simulink library "LibraryFM"  (R2016b)
settings: Solver=VariableStepAuto  StartTime=0.0  StopTime=10.0  RelTol=1e-3
undefined symbols (not defined in the file or in its folder): ActuatorStruct, drivePeakCurrent, FM1, Lb, Lf, Lu, motorTorqueConstant, RobotStruct, sampleTime, transmissionRatio
undefined symbols (not defined in the file): JointAbsoluteEncoderCounts_rev
libraries: simulink x34, LibraryFM x13, VariousBlocksLibrary x4, dspstat3 x1, simulink_extras x1, FM_Library x1
(part 3 of 3)

== matlab function LibraryFM/ToActuator1/DriveEnableLogic/8_JointVelocityGuard/LPF Diff/MATLAB Function ==
  data: u input; freq input; y output; y_prev input; sampleTime parameter
function y = fcn(u,freq,y_prev,sampleTime)
tau = 1/(freq*2*pi);
a = sampleTime/(sampleTime + tau);
y = y_prev*(1-a) + a*u;

== matlab function LibraryFM/Subsystem3/visuomotor rotation1 ==
  data: xBound input; pos_ref output; yBound input; vel input; pos_ref_prev input; sampleTime parameter; vel_ref output
function [pos_ref, vel_ref] = rotation(xBound, yBound, vel, pos_ref_prev,sampleTime)

persistent velDir;

if isempty(velDir)
    velDir = [1;0]; % initial velocity
end

pos_ref_tmp = pos_ref_prev + velDir*vel*sampleTime;

% check for x boundary
if (pos_ref_tmp(1) > xBound)
    velDir = [0;1];
elseif (pos_ref_tmp(1) < -xBound)
    velDir = [0;-1];
elseif (pos_ref_tmp(2) > yBound)
    velDir = [-1;0];
elseif (pos_ref_tmp(2) < -yBound)
    velDir = [1;0];
end

% forward Euler integration
pos_ref = pos_ref_prev + velDir*vel*sampleTime;
vel_ref = velDir*vel;

end

== matlab function LibraryFM/visuomotor rotation ==
  data: x_home input; x input; y output; theta input; doRotation input
function y = fcn(x_home,x,theta,doRotation)

x = x - x_home;

if (doRotation)
    R = [cos(theta) -sin(theta); 
         sin(theta) cos(theta)];
    y = R*x;
else
    y = x;
end

y = y + x_home;

== matlab function LibraryFM/DriveEnableLogic1/8_JointVelocityGuard/LPF Diff/MATLAB Function ==
  data: u input; freq input; y output; y_prev input; sampleTime parameter
function y = fcn(u,freq,y_prev,sampleTime)
tau = 1/(freq*2*pi);
a = sampleTime/(sampleTime + tau);
y = y_prev*(1-a) + a*u;

== stateflow chart LibraryFM/DriveEnableLogic1/DriveEnableStateMachine ==
  state Off
    state Par1 [parallel]
      settings: executionOrder=1
      state KeepLatchValue
      state ResetLatchValue
        en:
        LatchDriveError_Rising = 0;
      (default) -> KeepLatchValue
      KeepLatchValue -> ResetLatchValue : [after(10,msec)]
    state Par2 [parallel]
      settings: executionOrder=2
      state Off_NoErrorReset
        en:
        ControlWord = uint16(6);
      state Off_ErrorReset
        en:
        ControlWord = uint16(128+6);
      (default) -> Off_NoErrorReset
      Off_NoErrorReset -> Off_ErrorReset : [UseActuator && ...
          | AutoResetErrorInterval_Off_ms~=0 && ...
          |  after(AutoResetErrorInterval_Off_ms, msec)]
      Off_ErrorReset -> Off_NoErrorReset : [after(10,msec)]
  note: This can be either of states:
      | NotReadyToSwitchOn
      | SwitchOnDisabled
      | Fault
      | ReadyToSwitchOn
  note: This chart here  resembles the relevant parts of the DS402 specification on state transitions. Note however that I do NOT check which state the system is in by investigating the value of the StatusWord. Instead, I just assume that everything works as it should.
      |
      | (This chart evolved from a programmatic state machine which also did not do this)
  state ReadyToSwitchOn
  note: During this transition: Reset any error
  state SwitchedOn
    en: LatchDriveError_Rising=1;
    ex: LatchDriveError_Rising=0;
  note: We use this state also to reset the DriveError display.
  state OperationEnabled
    en:DriveShouldBeEnabled=1;
    ex:DriveShouldBeEnabled=0;
    state OE_NoErrorReset
      en:
      ControlWord = uint16(15);
    state OE_ErrorReset
      en:
      ControlWord = uint16(128+15);
    OE_ErrorReset -> OE_NoErrorReset : [after(10,msec)]
    (default) -> OE_NoErrorReset
    OE_NoErrorReset -> OE_ErrorReset : [AutoResetErrorInterval_On_ms~=0 && ...
        |  after(AutoResetErrorInterval_On_ms, msec)]
  (default) -> Off : {ControlWord=uint16(6)}
  (junction 41) -> Off : {ControlWord=uint16(6); ...
      | LatchDriveError_Rising=1}
  (junction 40) -> (junction 41)
  Off -> ReadyToSwitchOn : [UseActuator && EnableRequest]{ControlWord = uint16(128+6)}
  OperationEnabled -> ReadyToSwitchOn [order 2] : [EnableRequest]{ControlWord=uint16(128+6)}
  ReadyToSwitchOn -> (junction 22) : [after(20,msec)]
  (junction 22) -> (junction 40) [order 2] : [DriveErrorIn]
  (junction 44) -> (junction 40)
  (junction 22) -> SwitchedOn [order 1] : [~DriveErrorIn]{ControlWord=uint16(7)}
  SwitchedOn -> (junction 44) [order 2] : [~UseActuator || ...
      | DriveErrorIn || ...
      | DisableRequest]
  (junction 45) -> (junction 44)
  SwitchedOn -> OperationEnabled [order 1] : [after(150,msec)]{ControlWord=uint16(15)}
  OperationEnabled -> (junction 45) [order 1] : [~UseActuator || ...
      | DriveErrorIn || ...
      | DisableRequest]
  data: EnableRequest input; DisableRequest input; UseActuator input; DriveErrorIn input; ControlWord output uint16; DriveShouldBeEnabled output; AutoResetErrorInterval_Off_ms input; AutoResetErrorInterval_On_ms input; LatchDriveError_Rising output

== matlab function LibraryFM/StateMachineLocal/CheckVelThreshold ==
  data: qdot input; velBelowThreshold output; threshold input
function velBelowThreshold = checkVelThreshold(qdot, threshold)

velBelowThreshold = all(abs(qdot) <= threshold);

== matlab function LibraryFM/Admittance_BROS1/Virtual model ==
  data: lim_pos output; lim_vel output; lim_acc output; x1 output size=[2 1]; xdot1 output; xddot1 output; M_v input; B_v input; F input; x1_prev input size=2; xdot1_prev input size=2
function [lim_pos,lim_vel,lim_acc,x1,xdot1,xddot1] = AC(M_v, B_v, F, x1_prev, xdot1_prev)

Ts = 0.001;
maxRadius = 0.1;
maxVel = 2.0;
maxAcc = 100.0;

% lower bounds to 
m_v = max(0.2,M_v); %lower bound M_v = 1 kg
b_v = max(0,B_v);

% semi-implicit Euler integration
xddot1 = (F - b_v*xdot1_prev)/m_v;
[xddot1, lim_acc] = limit(xddot1,maxAcc);

xdot1 = xdot1_prev + xddot1*Ts;
[xdot1,lim_vel] = limit(xdot1,maxVel);

if (lim_vel)
    xddot1 = [0;0];
end

x1 = x1_prev + xdot1*Ts;
[x1,lim_pos] = limit(x1,maxRadius);
if (lim_pos)
    unitVec = x1/norm(x1);
    xdot1 = xdot1 - dot(unitVec,xdot1)*unitVec;     % remove normal component
    xddot1 = xddot1 - dot(unitVec,xddot1)*unitVec;  % remove normal component
end

end

function [y,lim] = limit(x,maxVal)
    vecLen = norm(x);
    if vecLen > maxVal
        y = x / vecLen * maxVal;
        lim = 1; 
    else
        y = x;
        lim = 0;
    end
end

== matlab function LibraryFM/FOAW1 ==
  data: x input; xdot output; sampleTime parameter; noise input
function xdot = foaw(x, sampleTime, noise)
%#codegen

SIZE = 200; % number of samples in buffer
NOISE = noise;
Ts = sampleTime;

persistent posbuffer;
persistent buffercntr;

% initialize buffer
if isempty(posbuffer)
    posbuffer = zeros(SIZE,1); % 1D case for now
    buffercntr = 0;
end

% fill buffer: shift data and add new value (loose oldest sample)
posbuffer = [posbuffer(2:end); x];
buffercntr = buffercntr + 1;
if buffercntr > SIZE, buffercntr = SIZE; end;

% if buffercntr = 1, only 1 data point is available, and you can't make a
% velocity prediction based on 1 data point. Set velocity ot 0, and return
% function
xdot = 0;
if buffercntr <= 3
    return;
end

for n = 2:2:buffercntr-1 % n = window size
        
    % step 2
    currentpos = posbuffer(end);

    % step 3 - calculate LS approximation of slope (hence velocity)
    b = n*sum(posbuffer(end-n:end)) - 2*sum(posbuffer(end-n:end).*(n:-1:0)');
    b = b / (Ts*n*(n+1)*(n+2)/6);

    % step 4 - check whether the line an + bn*Ts passes through all points inside the 
    % window within the uncertainty band of each point 
    jj = 0:n;
    yk_hat = currentpos-(b*jj*Ts);
    yk = posbuffer(end-jj)';
    if any(abs(yk_hat-yk) > NOISE)
        break;
    end

    xdot = b;
end

== matlab function LibraryFM/ToActuator1/DriveEnableLogic/EnableLogicDrive/enableDrive (CoE) ==
  data: ControlWord output; enable input; TimePerState_ms input
function ControlWord = enabledrive(enable, TimePerState_ms)
%#codegen
%
% Input arguments:
% enable:
%   0: Disable drive
%   Any non-zero: enable drive.
% TimePerState_ms:
%   A four-element array containing the time in ms for each state (states
%   are: 0, 128, 6, 7. The final state, 15, is kept until drive needs to be
%   disabled again.
%
% Changing enable forces the initialize-sequence to run
persistent previousEnable;
persistent counter;
if isempty(previousEnable)
    previousEnable = enable; % No enabling of the drive at startup
    counter = 1e6;
end;

if enable~=previousEnable
    counter = 0;
end;
previousEnable = enable;

TimePerState_cum = cumsum(TimePerState_ms);

if enable~=0
    counter = counter+1;
    if counter < TimePerState_cum(1);
        ControlWord_ = 0;
    elseif counter < TimePerState_cum(2);
        ControlWord_ = 128;
    elseif counter < TimePerState_cum(3);
        ControlWord_ = 6;
    elseif counter < TimePerState_cum(4);
        ControlWord_ = 7;
    else
        ControlWord_ = 15;
    end
else
    ControlWord_ = 6;
end

ControlWord = uint16(ControlWord_);

== matlab function LibraryFM/ToActuator1/EncodeDesiredTorque ==
  data: MotorTorque_Des_IU output int16; JointTorque_Des_Nm input; transmissionRatio parameter; motorTorqueConstant parameter; drivePeakCurrent parameter
function MotorTorque_Des_IU = EncodeDesiredTorque(JointTorque_Des_Nm, transmissionRatio, motorTorqueConstant, drivePeakCurrent)
%#codegen
% Calculate the target torque in incremental units for a desired joint
% torque.

% compute torque at motor (negate because sign change due to transmission)
torque_motor = JointTorque_Des_Nm / transmissionRatio; 

% desired current (i_des) = torque_motor / kt (torque constant)
i_des = torque_motor / motorTorqueConstant;

% calculate the target torque in incremental units [IU], see CoE manual
% Technosoftmotion
MotorTorque_Des_IU = int16( 65520*i_des / (2*drivePeakCurrent) );

== matlab function LibraryFM/FromActuator1/CalculateJointVelocity/FOAW ==
  data: x input; xdot output; sampleTime parameter; noise input
function xdot = foaw(x, sampleTime, noise)
%#codegen

SIZE = 100; % number of samples in buffer
NOISE = noise;
Ts = sampleTime;

persistent posbuffer;
persistent buffercntr;

% initialize buffer
if isempty(posbuffer)
    posbuffer = zeros(SIZE,1); % 1D case for now
    buffercntr = 0;
end

% fill buffer: shift data and add new value (loose oldest sample)
posbuffer = [posbuffer(2:end); x];
buffercntr = buffercntr + 1;
if buffercntr > SIZE, buffercntr = SIZE; end;

% if buffercntr = 1, only 1 data point is available, and you can't make a
% velocity prediction based on 1 data point. Set velocity ot 0, and return
% function
xdot = 0;
if buffercntr <= 3
    return;
end

for n = 1:buffercntr-1 % n = window size
        
    % step 2
    currentpos = posbuffer(end);

    % step 3 - calculate LS approximation of slope (hence velocity)
    b = n*sum(posbuffer(end-n:end)) - 2*sum(posbuffer(end-n:end).*(n:-1:0)');
    b = b / (Ts*n*(n+1)*(n+2)/6);

    % step 4 - check whether the line an + bn*Ts passes through all points inside the 
    % window within the uncertainty band of each point 
    jj = 0:n;
    yk_hat = currentpos-(b*jj*Ts);
    yk = posbuffer(end-jj)';
    if any(abs(yk_hat-yk) > NOISE)
        break;
    end

    xdot = b;
end

== matlab function LibraryFM/FromActuator1/CalibrateAbsEncoder ==
  data: encoderPosition input; JointPosition_AbsEnc_rad output; offset input
function JointPosition_AbsEnc_rad = CalibrateAbsoluteEncoder(encoderPosition, offset)
%#codegen

% unwrap encoder angle (in case the encoder goes through 0
% encoderPosition = unwrap(encoderPosition);
encoderPosition = encoderPosition;

% remove offset
JointPosition_AbsEnc_rad = encoderPosition - offset;

% since the absolute encoder is mounted upside-down, negate the
% jointposition angle
JointPosition_AbsEnc_rad = -JointPosition_AbsEnc_rad;

== matlab function LibraryFM/FromActuator1/CalibrateIncEncoder     ==
  data: JointPosition_IncEnc_rad output; MotorPosition_rad input; MotorPositionCalibrated_rad output; transmissionRatio parameter; Calibrate input; JointPosition_AbsEnc_rad input
function [JointPosition_IncEnc_rad,MotorPositionCalibrated_rad]...
    = CalibrateIncEncoder( MotorPosition_rad,transmissionRatio, Calibrate,JointPosition_AbsEnc_rad)
%#codegen

% This block includes calibration such that (ideally) the motor angle is
% zero when the joint angle and spring deflection are zero as well. Before
% the calibration has occurred, the output of this function is -1e9*. This
% is chosen such that the value is always outside the allowed motor angle
% range; this prevents the drive from being allowed to turn on.
% 
% * I wanted to use -inf as starting function, but I'm not sure whether
%   that will be handled correctly in all cases.

persistent isCalibrated;
persistent offset;

if isempty(isCalibrated) % no calibration needed
    isCalibrated = 0;
    offset = 0;
end;


if Calibrate && ~isCalibrated
%     if ~isempty(JointPosition_AbsEnc_rad)
        target_pos_mot_rad = transmissionRatio * JointPosition_AbsEnc_rad; % This is what we should read
%         target_pos_mot_rad = CalibrationAngle; % This is what we should read / fix for now
        offset = target_pos_mot_rad - MotorPosition_rad; % calculate offset
%     else
%         % no absolute encoder data available, offset is zero
%         offset = 0;
%     end
    isCalibrated = 1;
end;

% if already calibrated, calculate calibrated motor angle
if isCalibrated
    MotorPositionCalibrated_rad = MotorPosition_rad + offset;
    JointPosition_IncEnc_rad = MotorPositionCalibrated_rad / transmissionRatio;
else
    MotorPositionCalibrated_rad = MotorPosition_rad;
    JointPosition_IncEnc_rad = MotorPositionCalibrated_rad / transmissionRatio;
end;

== matlab function LibraryFM/FromActuator1/CheckOperationEnabled ==
  data: u input; y output
function y = fcn(u)
%#codegen

mask  = bin2dec('0000000001101111');
match = bin2dec('0000000000100111');

masked = bitand(u,mask);
if masked==match
    y=1;
else
    y=0;
end;

== matlab function LibraryFM/StateMachineLocal/checkEndpointPosition ==
  data: x input; homeLocation input; isAtEndpoint output; threshold input
function isAtEndpoint = checkEndpointPosition(x, homeLocation, threshold)
% check whether the endpoint position is within a specified circle with
% radius threshold and midopoint HomePosition

% calculate distance between home position and joint positions
d = sqrt(sum((homeLocation - x).^2));

if imag(d) || isinf(d) || isnan(d)
    isAtEndpoint = false;
else
    isAtEndpoint = (d <= threshold);
end

== matlab function LibraryFM/DataFromEtherCAT/FTSensor_K6D27/SensorToOperationalSpace ==
  data: q_all input; Fs input; FTOpSpace output; transmatside input
function FTOpSpace = ForceSensorToOperationalSpace(q_all,Fs,transmatside)
%#codegen
q1 = q_all(1);
q2 = q_all(2);
q4 = q_all(4);
q5 = q_all(5);

% based on which arm the force sensor is connected
switch transmatside
    case 1
        alpha = pi-q2;   
        beta = q1+alpha-pi/2;
        R0 = rotmat(beta);
        R = blkdiag(R0,R0); % transform forces and moments
    case 2
        alpha = -(pi - q4);
        beta = q5+alpha-pi/2;
        R0 = rotmat(beta);
        R = blkdiag(R0,R0); % transform forces and moments
    otherwise
        R = eye(length(Fs));
end

% transform force
FTOpSpace = R*Fs;

function R = rotmat(q)

R = [cos(q) -sin(q) 0;...
      sin(q)  cos(q) 0;...
      0       0      1];

== matlab function LibraryFM/DataToEtherCAT/WorkspacePositionGuard/CheckForSingularity ==
  data: J input; kappa output
function kappa = conditionnumber(J)
%#codegen

kappa = norm(pinv(J))*norm(J);

== matlab function LibraryFM/DataToEtherCAT/WorkspacePositionGuard/CheckInternalAngles ==
  data: theta input; angleError output
function angleError = checkInternalErrors(theta)
%#codegen

angleError = 0;
if any(theta([2 4]) >= 0.95*pi)
    angleError = 1;
end

== matlab function LibraryFM/DataToEtherCAT/WorkspacePositionGuard/EndpointPositionGuard ==
  data: xe input; error output; correctState input
function error = fcn(xe, correctState)
%#codegen


error = 0;

% only check workspace boundaries after homing state is done
if ~correctState 
    return; 
end

% x0 = 0;
% y0 = 0.2354;
% a = 0.11;
% b = 0.08;

% workspace (see design document)
x0 = 0;
y0 = 0.25024;
a = 0.1746;
b = 0.13;%0.1048;

% check if endpoint is outside a predefined ellipse
x = xe(1);
y = xe(2);

% workspace is defined as an ellipse
e = (x-x0)^2 / a^2 + (y-y0)^2 / b^2;

% if is larger than 1, the endpoint is outside the workspace
if e > 1
    error = 1;
end

== matlab function LibraryFM/FromActuator1/DecodeActualTorque ==
  data: JointTorque_Act_Nm output; MotorCurrent_Act_IU input int16; transmissionRatio parameter; drivePeakCurrent parameter; motorTorqueConstant parameter
function JointTorque_Act_Nm = DecodeActualTorque(MotorCurrent_Act_IU, transmissionRatio, drivePeakCurrent, motorTorqueConstant)
%#codegen
%

% convert incremental units to motor torque value. See the technosoft CoE
% manual for the decoding
torquemotor_act = motorTorqueConstant * (double(MotorCurrent_Act_IU)*2*drivePeakCurrent / 65520);

% motor torque to joint torque (transmission). Negate due to sign change
% due to transmission.
JointTorque_Act_Nm = torquemotor_act * transmissionRatio;

== matlab function LibraryFM/FromActuator1/DecodeEncoder_AbsEnc ==
  data: Encoder_counts input; EncoderCounts_rev parameter; EncoderPosition_rad output
function EncoderPosition_rad = ...
    DecodeEncoder(Encoder_counts, EncoderCounts_rev)
%#codegen

% This block decodes the motor encoder counts to the motor angle

EncoderPosition_rad = (double(Encoder_counts) / EncoderCounts_rev * 2 * pi);

== matlab function LibraryFM/FromActuator1/DecodeEncoder_IncEnc ==
  data: Encoder_counts input; EncoderCounts_rev parameter; EncoderPosition_rad output
function EncoderPosition_rad = ...
    DecodeEncoder(Encoder_counts, EncoderCounts_rev)
%#codegen

% This block decodes the motor encoder counts to the motor angle

EncoderPosition_rad = (double(Encoder_counts) / EncoderCounts_rev * 2 * pi);
